simulink model "modello_completo_simulink2017b"  (R2017b)
settings: Solver=VariableStepAuto  StartTime=0.0  StopTime=10  RelTol=1e-3
undefined symbols (not defined in the file): a1, a2, AHRS_bias, AHRS_sample_time, AHRS_var, alpha1, alpha2, c, current, D, dead_zone_limit, DVL_sample_t, DVL_var1, DVL_var2, DVL_var3, gps_sample_t, IMU_sample_time, initial, M, M_inv, n_max, omega, ps_sample_t, ps_sample_t2, ps_var, ps_var2, pylonCenter, pylonRadius, rho, s_data, TAM
libraries: simulink x3
(part 2 of 2)

== system modello_completo_simulink2017b/Vehicle Model/Thrusters/T/Thruster 4 ==
  note: n is the rotational speed of the thruster
      | V is the speed component of the water along the thruster axis
      |
      | n is saturated according to data
      | a dead zone is considered according to data
      | the thruster is characterised by 1st order dynamics (tau = 0.2s)
  n [rad/s] : Inport
  V [m/s] : Inport  Port=2
  Dead Zone : DeadZone  LowerValue=-dead_zone_limit  UpperValue=dead_zone_limit  SaturateOnIntegerOverflow=on
  MATLAB Function : MATLAB Function  TreatAsAtomicUnit=on
  Saturation : Saturate  UpperLimit=n_max  LowerLimit=-n_max
  Transfer Fcn : TransferFcn  Denominator=[0.2 1]
  T i : Outport
  wires:
  V [m/s]/1 -> MATLAB Function/2(V)
  Saturation/1 -> MATLAB Function/1(n)
  Transfer Fcn/1 -> Saturation/1
  Dead Zone/1 -> Transfer Fcn/1
  n [rad/s]/1 -> Dead Zone/1
  MATLAB Function/1(T) -> T i/1

== system modello_completo_simulink2017b/Vehicle Model/Thrusters/T/Thruster 5 ==
  note: n is the rotational speed of the thruster
      | V is the speed component of the water along the thruster axis
      |
      | n is saturated according to data
      | a dead zone is considered according to data
      | the thruster is characterised by 1st order dynamics (tau = 0.2s)
  n [rad/s] : Inport
  V [m/s] : Inport  Port=2
  Dead Zone : DeadZone  LowerValue=-dead_zone_limit  UpperValue=dead_zone_limit  SaturateOnIntegerOverflow=on
  MATLAB Function : MATLAB Function  TreatAsAtomicUnit=on
  Saturation : Saturate  UpperLimit=n_max  LowerLimit=-n_max
  Transfer Fcn : TransferFcn  Denominator=[0.2 1]
  T i : Outport
  wires:
  V [m/s]/1 -> MATLAB Function/2(V)
  Saturation/1 -> MATLAB Function/1(n)
  Transfer Fcn/1 -> Saturation/1
  Dead Zone/1 -> Transfer Fcn/1
  n [rad/s]/1 -> Dead Zone/1
  MATLAB Function/1(T) -> T i/1

== system modello_completo_simulink2017b/Vehicle Model/Thrusters/T/Thruster 6 ==
  note: n is the rotational speed of the thruster
      | V is the speed component of the water along the thruster axis
      |
      | n is saturated according to data
      | a dead zone is considered according to data
      | the thruster is characterised by 1st order dynamics (tau = 0.2s)
  n [rad/s] : Inport
  V [m/s] : Inport  Port=2
  Dead Zone : DeadZone  LowerValue=-dead_zone_limit  UpperValue=dead_zone_limit  SaturateOnIntegerOverflow=on
  MATLAB Function : MATLAB Function  TreatAsAtomicUnit=on
  Saturation : Saturate  UpperLimit=n_max  LowerLimit=-n_max
  Transfer Fcn : TransferFcn  Denominator=[0.2 1]
  T i : Outport
  wires:
  V [m/s]/1 -> MATLAB Function/2(V)
  Saturation/1 -> MATLAB Function/1(n)
  Transfer Fcn/1 -> Saturation/1
  Dead Zone/1 -> Transfer Fcn/1
  n [rad/s]/1 -> Dead Zone/1
  MATLAB Function/1(T) -> T i/1

== system modello_completo_simulink2017b/Vehicle Model/Thrusters/T/Thruster 7 ==
  note: n is the rotational speed of the thruster
      | V is the speed component of the water along the thruster axis
      |
      | n is saturated according to data
      | a dead zone is considered according to data
      | the thruster is characterised by 1st order dynamics (tau = 0.2s)
  n [rad/s] : Inport
  V [m/s] : Inport  Port=2
  Dead Zone : DeadZone  LowerValue=-dead_zone_limit  UpperValue=dead_zone_limit  SaturateOnIntegerOverflow=on
  MATLAB Function : MATLAB Function  TreatAsAtomicUnit=on
  Saturation : Saturate  UpperLimit=n_max  LowerLimit=-n_max
  Transfer Fcn : TransferFcn  Denominator=[0.2 1]
  T i : Outport
  wires:
  V [m/s]/1 -> MATLAB Function/2(V)
  Saturation/1 -> MATLAB Function/1(n)
  Transfer Fcn/1 -> Saturation/1
  Dead Zone/1 -> Transfer Fcn/1
  n [rad/s]/1 -> Dead Zone/1
  MATLAB Function/1(T) -> T i/1

== matlab function modello_completo_simulink2017b/Vehicle Model/Model Vehicle/D ==
  data: ni_r input; F_d output; rho input
function F_d = D_forces(ni_r, rho)
    ni_lin = ni_r(1:3);
    ni_ang = ni_r(4:6);
    a = 0.35;
    b = a;
    c = 0.19;
    A_ab = pi*a*b;      % moto lin lungo z; rotatorio intorno a x e y
    A_bc = pi*b*c;      % moto lin lungo x; rotatorio intorno a z
    A_ac = pi*a*c;      % moto lin lungo y
%     C_d  =  0.0489;
%     D_coeff = -1/2*rho*C_d*diag([A_bc, A_ac, A_ab, A_bc, A_ac, A_ab]);
%     F_d = D_coeff*(abs(ni_r).*ni_r);
    visc = 0.001;       % Pa*s (per una temperatura di 20° e rho = 1030)
    vmax = 0.3;
    Di = 0.7;
    Re = Di/(visc/rho)*vmax; % Re = 2*1e5
    Cd = 0.49;
    rm_z = 4*c/(3*pi);
    rm_xy = 4*a/(3*pi);
    D_lin = -1/2*rho*Cd*diag([A_bc, A_ac, A_ab])*(abs(ni_lin).*ni_lin);
    D_ang = -1/2*rho*Cd*diag([rm_xy^3*A_ab, rm_xy^3*A_ab, rm_z^3*A_bc])*(abs(ni_ang).*ni_ang);
    F_d = [D_lin; D_ang];
end

== matlab function modello_completo_simulink2017b/Vehicle Model/Model Vehicle/C ==
  data: ni_r input; F_c output; M input
function F_c = C(ni_r, M)
    ni = ni_r;
    M11 = M(1:3,1:3);
    M22 = M(4:6,4:6);
    ni1 = ni(1:3);
    ni2 = ni(4:6);
    C11 = zeros(3,3);
    s1 = M11*ni1;
    C12 = - [0 -s1(3) s1(2); s1(3) 0 -s1(1); -s1(2) s1(1) 0];
    C21 = C12;
    s2 = M22*ni2;
    C22 = - [0 -s2(3) s2(2); s2(3) 0 -s2(1); -s2(2) s2(1) 0];
    F_c = [C11 C12; C21 C22]*ni_r;
end

== matlab function modello_completo_simulink2017b/Vehicle Model/Model Vehicle/grav ==
  data: rho input; eta input; F_g output
function F_g = grav(rho, eta)
    eta2 = eta(4:6);
    g = 9.81;   
    a = 0.35;
    b = a;
    c = 0.19;
    massa = 100;
    if eta(3) >= c
       V = 4/3*pi*a*b*c;
    else
       V = 4/3*pi*a*b*c - (pi*a*b/(3*c^2))*((eta(3)-c)^2)*(3*c - abs(eta(3) - c)); 
    end
    W = massa*g;
    B = rho*V*g;
    J = Jac(eta2);
    J1 = J(1:3,1:3);
    J2 = J(4:6,4:6);
    f_g = inv(J1)*[0; 0; W];
    f_b = inv(J1)*[0; 0; -B];
    r_g = [0; 0; 0];
    r_b = [0; 0; -c/2];
    %TODO: inserire un contributo nullo di forza quando siamo a galla (?)
%     if eta(3) < 0
%        F_g = [0; 0; 0; 0; 0; 0];
%     else
    F_g = -[f_g + f_b; cross(r_g,f_g) + cross(r_b,f_b)];
%     end
end

== matlab function modello_completo_simulink2017b/Vehicle Model/Model Vehicle/Kinematic/Jac ==
  data: eta input; J output
function J = Jac(eta)
    eta2 = eta(4:6);
    phi = eta2(1);
    theta = eta2(2);
    psi = eta2(3);
    Rx = [1 0 0; 0 cos(phi) sin(phi); 0 -sin(phi) cos(phi)];
    Ry = [cos(theta) 0 -sin(theta); 0 1 0; sin(theta) 0 cos(theta)];
    Rz = [cos(psi) sin(psi) 0; -sin(psi) cos(psi) 0; 0 0 1];
    J1 = Rz'*Ry'*Rx';
    J2 = [1 sin(phi)*tan(theta) cos(phi)*tan(theta); ...
        0 cos(phi) -sin(phi); ...
        0 sin(phi)/cos(theta) cos(phi)/cos(theta)];
    J = blkdiag(J1, J2);
end

== matlab function modello_completo_simulink2017b/Vehicle Model/Thrusters/T/Thruster 1/MATLAB Function ==
  data: n input; T output; V input; D parameter; omega parameter; a1 parameter; a2 parameter; alpha1 parameter; alpha2 parameter
function T = thrusterModel(n, V, D, omega, a1, a2, alpha1, alpha2)

Va = (1-omega) * V;     % Advancement velocity at the propeller
J0 = Va/(n*D);          % Advancement Coefficient

if J0 > -alpha1/alpha2  % Out of linearity domain (right side)
    T = 0;              % A null generated thrust is assumed
    
elseif J0 < 0           % Out of linearity domain (left side)
    T = a1*abs(n)*n;    % Bollard thrust is assumed

else                    % Within the linearity domain
    T = a1*abs(n)*n - a2*abs(n)*V;
end

== matlab function modello_completo_simulink2017b/Vehicle Model/Thrusters/T/Thruster 2/MATLAB Function ==
  data: n input; T output; V input; D parameter; omega parameter; a1 parameter; a2 parameter; alpha1 parameter; alpha2 parameter
function T = thrusterModel(n, V, D, omega, a1, a2, alpha1, alpha2)

Va = (1-omega) * V;     % Advancement velocity at the propeller
J0 = Va/(n*D);          % Advancement Coefficient

if J0 > -alpha1/alpha2  % Out of linearity domain (right side)
    T = 0;              % A null generated thrust is assumed
    
elseif J0 < 0           % Out of linearity domain (left side)
    T = a1*abs(n)*n;    % Bollard thrust is assumed

else                    % Within the linearity domain
    T = a1*abs(n)*n - a2*abs(n)*V;
end

== matlab function modello_completo_simulink2017b/Vehicle Model/Thrusters/T/Thruster 3/MATLAB Function ==
  data: n input; T output; V input; D parameter; omega parameter; a1 parameter; a2 parameter; alpha1 parameter; alpha2 parameter
function T = thrusterModel(n, V, D, omega, a1, a2, alpha1, alpha2)

Va = (1-omega) * V;     % Advancement velocity at the propeller
J0 = Va/(n*D);          % Advancement Coefficient

if J0 > -alpha1/alpha2  % Out of linearity domain (right side)
    T = 0;              % A null generated thrust is assumed
    
elseif J0 < 0           % Out of linearity domain (left side)
    T = a1*abs(n)*n;    % Bollard thrust is assumed

else                    % Within the linearity domain
    T = a1*abs(n)*n - a2*abs(n)*V;
end

== matlab function modello_completo_simulink2017b/Vehicle Model/Thrusters/T/Thruster 4/MATLAB Function ==
  data: n input; T output; V input; D parameter; omega parameter; a1 parameter; a2 parameter; alpha1 parameter; alpha2 parameter
function T = thrusterModel(n, V, D, omega, a1, a2, alpha1, alpha2)

Va = (1-omega) * V;     % Advancement velocity at the propeller
J0 = Va/(n*D);          % Advancement Coefficient

if J0 > -alpha1/alpha2  % Out of linearity domain (right side)
    T = 0;              % A null generated thrust is assumed
    
elseif J0 < 0           % Out of linearity domain (left side)
    T = a1*abs(n)*n;    % Bollard thrust is assumed

else                    % Within the linearity domain
    T = a1*abs(n)*n - a2*abs(n)*V;
end

== matlab function modello_completo_simulink2017b/Vehicle Model/Thrusters/T/Thruster 5/MATLAB Function ==
  data: n input; T output; V input; D parameter; omega parameter; a1 parameter; a2 parameter; alpha1 parameter; alpha2 parameter
function T = thrusterModel(n, V, D, omega, a1, a2, alpha1, alpha2)

Va = (1-omega) * V;     % Advancement velocity at the propeller
J0 = Va/(n*D);          % Advancement Coefficient

if J0 > -alpha1/alpha2  % Out of linearity domain (right side)
    T = 0;              % A null generated thrust is assumed
    
elseif J0 < 0           % Out of linearity domain (left side)
    T = a1*abs(n)*n;    % Bollard thrust is assumed

else                    % Within the linearity domain
    T = a1*abs(n)*n - a2*abs(n)*V;
end

== matlab function modello_completo_simulink2017b/Vehicle Model/Thrusters/T/Thruster 6/MATLAB Function ==
  data: n input; T output; V input; D parameter; omega parameter; a1 parameter; a2 parameter; alpha1 parameter; alpha2 parameter
function T = thrusterModel(n, V, D, omega, a1, a2, alpha1, alpha2)

Va = (1-omega) * V;     % Advancement velocity at the propeller
J0 = Va/(n*D);          % Advancement Coefficient

if J0 > -alpha1/alpha2  % Out of linearity domain (right side)
    T = 0;              % A null generated thrust is assumed
    
elseif J0 < 0           % Out of linearity domain (left side)
    T = a1*abs(n)*n;    % Bollard thrust is assumed

else                    % Within the linearity domain
    T = a1*abs(n)*n - a2*abs(n)*V;
end

== matlab function modello_completo_simulink2017b/Vehicle Model/Thrusters/T/Thruster 7/MATLAB Function ==
  data: n input; T output; V input; D parameter; omega parameter; a1 parameter; a2 parameter; alpha1 parameter; alpha2 parameter
function T = thrusterModel(n, V, D, omega, a1, a2, alpha1, alpha2)

Va = (1-omega) * V;     % Advancement velocity at the propeller
J0 = Va/(n*D);          % Advancement Coefficient

if J0 > -alpha1/alpha2  % Out of linearity domain (right side)
    T = 0;              % A null generated thrust is assumed
    
elseif J0 < 0           % Out of linearity domain (left side)
    T = a1*abs(n)*n;    % Bollard thrust is assumed

else                    % Within the linearity domain
    T = a1*abs(n)*n - a2*abs(n)*V;
end

== matlab function modello_completo_simulink2017b/Vehicle Model/Model Vehicle/MATLAB Function ==
  data: coord_pylon input; eta input; eta_ecef output
function eta_ecef = nedToEcef(coord_pylon, eta)

    coder.extrinsic('wgs84Ellipsoid');

    coder.extrinsic('ned2geodetic');
    
    eta_pos = eta(1:6);
    wgs84 = wgs84Ellipsoid('meter'); %TODO verificare che esprima le coordinate nello stesso modo dell'ECEF dato in missionB.m
    [eta_pos(1), eta_pos(2)] = ned2geodetic(eta(1), eta(2), eta(3), coord_pylon(1), coord_pylon(2), coord_pylon(3), wgs84,'degrees');
    
    eta_pos(3) = eta(3);
    eta_pos(4:6) = eta_pos(4:6);
    
    eta_ecef = eta_pos;
    
end

== matlab function modello_completo_simulink2017b/Vehicle Model/MATLAB Function ==
  data: eta input; ni_c output; current input
function ni_c = current_ned2body(eta, current)
    eta2 = eta(4:6)*pi/180;     % eta2 espresso in radianti
    ni_c = Jac(eta2)'*current;
end

== matlab function modello_completo_simulink2017b/Vehicle Model/Thrusters/T/MATLAB Function ==
  data: ni input; v_th output
function v_th = thrusters(ni)
p1 = [-0.35 -0.25 0]';
p2 = [-0.35 0.25 0]';
p3 = [-0.25 -0.35 0]';
p4 = [0.25 0.35 0]';
p5 = [-0.25 -0.25 -0.19]';
p6 = [-0.25 0.25 -0.19]';
p7 = [0.25 0 -0.19]';

t1 = [1 0 0]';
t2 = t1;
t3 = [0 1 0]';
t4 = -t3;
t5 = [0 0 1]';
t6 = t5;
t7 = t5;

v_lin = ni(1:3);
v_ang = ni(4:6);

vp1 = v_lin + cross(v_ang, p1);
vp2 = v_lin + cross(v_ang, p2);
vp3 = v_lin + cross(v_ang, p3);
vp4 = v_lin + cross(v_ang, p4);
vp5 = v_lin + cross(v_ang, p5);
vp6 = v_lin + cross(v_ang, p6);
vp7 = v_lin + cross(v_ang, p7);

v1 = vp1'*t1;
v2 = vp2'*t2;
v3 = vp3'*t3;
v4 = vp4'*t4;
v5 = vp5'*t5;
v6 = vp6'*t6;
v7 = vp7'*t7;

v_th = [ v1 v2 v3 v4 v5 v6 v7]';
end

== matlab function modello_completo_simulink2017b/Vehicle Model/Thrusters/saturation_tau ==
  data: tau input; tau_sat output; eta input
function tau_sat = sat_tau(tau, eta)
    tau_sat = [0;0;0;0;0;0];
    tau_sat = tau;

    if eta(3) < 0.1 %semiasse c
        tau_sat(3) = 0;
    end
    
end

== matlab function modello_completo_simulink2017b/Navigation/Geodetic to NED/MATLAB Function2 ==
  data: GPS_geodetic input; GPS_flag input; GPS_NED output; depth input; pylonCenter parameter
function GPS_NED = Geo2NED(GPS_geodetic, GPS_flag, depth, pylonCenter)

if GPS_flag == 0
    GPS_NED = [0;0;0];
    return
end

%% variabili

phi = GPS_geodetic(1);
lambda = GPS_geodetic(2);
h = -depth;

phi_pyl = pylonCenter(1) * pi/180;    % GPS_geodetic_origin 
lambda_pyl = pylonCenter(2) * pi/180;

% r_e = 6378137;
% epsilon = 0.08181919;
% N = r_e / (sqrt(1 - epsilon^2 * (sin(phi))^2));
% N_pyl = r_e / (sqrt(1 - epsilon^2 * (sin(phi_pyl))^2));
% 
% eta_ECEF_origin = zeros(3,1);
% eta_ECEF_origin = [(N_pyl + h) * cos(phi_pyl) * cos(lambda_pyl);
%                    (N_pyl + h) * cos(phi_pyl) * sin(lambda_pyl);
%                    (N_pyl*(1-epsilon^2) + h) * sin(phi_pyl)];
% 
% %% da geodetic a ECEF
% eta_ECEF_P = zeros(3,1);
% eta_ECEF_P = [(N + h) * cos(phi) * cos(lambda);
%               (N + h) * cos(phi) * sin(lambda);
%               (N*(1-epsilon^2) + h) * sin(phi)];
% 
% %% da ECEF a NED
% 
% R_ECEF_NED = [-sin(phi_pyl)*cos(lambda_pyl),    -sin(phi_pyl)*sin(lambda_pyl),  cos(phi_pyl);   % matrice "C" 3x3
%               -sin(lambda_pyl),                 cos(lambda_pyl),                0;
%               -cos(phi_pyl)*cos(lambda_pyl),    -cos(phi_pyl)*sin(lambda_pyl),  -sin(phi_pyl)];
% 
% R_ECEF_NED_2 = R_ECEF_NED(1:2,:);   % matrice "C" 2x3
% eta_NED_GPS = zeros(2,1);
% eta_ECEF = (eta_ECEF_P - eta_ECEF_origin);
% 
% eta_NED_GPS = R_ECEF_NED_2 * eta_ECEF;   % solo gli elementi x,y di eta
coder.extrinsic('wgs84Ellipsoid');

coder.extrinsic('geodetic2ned');
    
[x_gps2, y_gps2, z_gps2] = geodetic2ned(phi, lambda, -depth, phi_pyl, lambda_pyl, 0, wgs84Ellipsoid, 'radians');
eta_NED_GPS = [x_gps2; y_gps2];
GPS_NED = zeros(3,1);
GPS_NED(1) = eta_NED_GPS(1);
GPS_NED(2) = eta_NED_GPS(2);
GPS_NED(3) = GPS_flag;
                                                            % uscita in radianti

== matlab function modello_completo_simulink2017b/Navigation/MATLAB Function ==
  data: flag_depth input; flag_AHRS input; error_flag output; flag_DVL input; flag_sonar input
function error_flag = fcn(flag_depth, flag_AHRS, flag_DVL, flag_sonar)
flag_ahrs = flag_AHRS(1) & flag_AHRS(2) & flag_AHRS(3);
error_flag = flag_depth & flag_ahrs & flag_DVL & flag_sonar;
%se vi è un errore vale 0

== matlab function modello_completo_simulink2017b/Navigation/MATLAB Function7 ==
  data: eta2 output; lin_acc input; nu2 output; ang_vel input; orientation input
function [eta2, nu2]= AHRS_signals(lin_acc, ang_vel, orientation)
acc = lin_acc(1:3);
nu2 = ang_vel(1:3);
eta2 = orientation(1:3);

== matlab function modello_completo_simulink2017b/Navigation/MATLAB Function8 ==
  data: dvl input; velocity_est output; flag_DVL output
function [velocity_est, flag_DVL] = DVL_signals(dvl)
% y = lowpass(u, 0.01);
flag_DVL = dvl(4);
velocity_est = dvl(1:3);

== matlab function modello_completo_simulink2017b/Navigation/NED to Geodetic/MATLAB Function1 ==
  data: eta_NED input; eta_geodetic output; depth input; pylonCenter parameter
function eta_geodetic = NED2Geo(eta_NED, depth, pylonCenter)
coder.extrinsic('fcn_NED2GeoN');
eta_geodetic = [0; 0];
eta_geodetic = fcn_NED2GeoN(eta_NED, depth, pylonCenter);
end

== matlab function modello_completo_simulink2017b/Navigation/Relative estiamtion/Sonar trigger/MATLAB Function ==
  data: sonar input; sum input; pulse output; prev output
function [pulse, prev] = fcn(sonar, sum)


if all(sum) == 0
    pulse = 0;
else
    pulse = 1;
end

prev = sonar;

== matlab function modello_completo_simulink2017b/Navigation/Relative estiamtion/Subsystem/MATLAB Function9 ==
  data: sonar input; orientation input; distance output; alpha output; flag_sonar output; pylonRadius parameter
function [distance, alpha, flag_sonar] = relative_values(sonar, orientation, pylonRadius)
coder.extrinsic('fcn_sonar');
distance = 0;
alpha = 0;
flag_sonar = 0;
[distance, alpha, flag_sonar] = fcn_sonar(sonar, orientation, pylonRadius);
end

== matlab function modello_completo_simulink2017b/Navigation/Subsystem/EKF/EKF_depth/Correzione ==
  data: P_depth output; P_depth input; hat_depth input; depth_meas input; hat_depth output; flag_depth output; R parameter
function [P_depth, hat_depth, flag_depth]  = EKF_depth(P_depth, hat_depth, depth_meas, R)

%% Inizializzazione

DT = 1/50;                           % frequenza profondimetro = 50 Hz

%% EKF



% Correzione
z_tilde = depth_meas(1) - hat_depth;
H = 1;
S = H * P_depth * H' + R(3,3);

K = P_depth * H' * S^(-1);

hat_depth = hat_depth + K * z_tilde;   
P_depth   = (1 - K * H) * P_depth;  

    
flag_depth = depth_meas(2);

== matlab function modello_completo_simulink2017b/Navigation/Subsystem/EKF/EKF_depth/Predizione ==
  data: P_depth output; P_depth input; hat_depth input; dT input; hat_depth output; orientation input; dvl input; init_depth input; P0_depth input; ahrs_flag input; Q parameter
function [P_depth, hat_depth]  = EKF_depth(P_depth, hat_depth, dT, orientation, dvl, init_depth, P0_depth, ahrs_flag, Q)

%% Inizializzazione
                     % [s]  depth period
dvl_flag = dvl(4);

%coder.extrinsic('Lk_func');

if hat_depth == 0
    hat_depth = init_depth;
    P_depth = P0_depth;
end

if (ahrs_flag && dvl_flag) == 1

    phi    =  orientation(1);  % roll
    theta  =  orientation(2);  % pitch
    psi_    =  orientation(3);  % yaw
    vel    = [dvl(1); dvl(2); dvl(3)];
    J=zeros(3,3);
    Lk=zeros(3,6);
    
%    [J, Lk] = Lk_func(dT, psi, theta, psi, vel);

J = [ cos(psi_)*cos(theta), cos(psi_)*sin(phi)*sin(theta) - cos(phi)*sin(psi_), sin(phi)*sin(psi_) + cos(phi)*cos(psi_)*sin(theta);
       cos(theta)*sin(psi_), cos(phi)*cos(psi_) + sin(phi)*sin(psi_)*sin(theta), cos(phi)*sin(psi_)*sin(theta) - cos(psi_)*sin(phi);
         -sin(theta),                                cos(theta)*sin(phi),                                cos(phi)*cos(theta)];
     
%J = eval(subs(J1, {phi, theta, psi_}, {phi, theta, psi_}));

x = dvl(1);
y = dvl(2);
z = dvl(3);
n_ahrs1 = 0;
n_ahrs2 = 0;
n_ahrs3 = 0;

Lk = [  dT*(y*(sin(n_ahrs1 + phi)*sin(n_ahrs3 + psi_) + cos(n_ahrs1 + phi)*cos(n_ahrs3 + psi_)*sin(n_ahrs2 + theta)) + z*(cos(n_ahrs1 + phi)*sin(n_ahrs3 + psi_) - cos(n_ahrs3 + psi_)*sin(n_ahrs1 + phi)*sin(n_ahrs2 + theta))), dT*(z*cos(n_ahrs1 + phi)*cos(n_ahrs3 + psi_)*cos(n_ahrs2 + theta) - x*cos(n_ahrs3 + psi_)*sin(n_ahrs2 + theta) + y*cos(n_ahrs3 + psi_)*cos(n_ahrs2 + theta)*sin(n_ahrs1 + phi)), -dT*(y*(cos(n_ahrs1 + phi)*cos(n_ahrs3 + psi_) + sin(n_ahrs1 + phi)*sin(n_ahrs3 + psi_)*sin(n_ahrs2 + theta)) - z*(cos(n_ahrs3 + psi_)*sin(n_ahrs1 + phi) - cos(n_ahrs1 + phi)*sin(n_ahrs3 + psi_)*sin(n_ahrs2 + theta)) + x*cos(n_ahrs2 + theta)*sin(n_ahrs3 + psi_)), dT*cos(n_ahrs3 + psi_)*cos(n_ahrs2 + theta), -dT*(cos(n_ahrs1 + phi)*sin(n_ahrs3 + psi_) - cos(n_ahrs3 + psi_)*sin(n_ahrs1 + phi)*sin(n_ahrs2 + theta)),  dT*(sin(n_ahrs1 + phi)*sin(n_ahrs3 + psi_) + cos(n_ahrs1 + phi)*cos(n_ahrs3 + psi_)*sin(n_ahrs2 + theta));
 -dT*(y*(cos(n_ahrs3 + psi_)*sin(n_ahrs1 + phi) - cos(n_ahrs1 + phi)*sin(n_ahrs3 + psi_)*sin(n_ahrs2 + theta)) + z*(cos(n_ahrs1 + phi)*cos(n_ahrs3 + psi_) + sin(n_ahrs1 + phi)*sin(n_ahrs3 + psi_)*sin(n_ahrs2 + theta))), dT*(z*cos(n_ahrs1 + phi)*cos(n_ahrs2 + theta)*sin(n_ahrs3 + psi_) - x*sin(n_ahrs3 + psi_)*sin(n_ahrs2 + theta) + y*cos(n_ahrs2 + theta)*sin(n_ahrs1 + phi)*sin(n_ahrs3 + psi_)),  dT*(z*(sin(n_ahrs1 + phi)*sin(n_ahrs3 + psi_) + cos(n_ahrs1 + phi)*cos(n_ahrs3 + psi_)*sin(n_ahrs2 + theta)) - y*(cos(n_ahrs1 + phi)*sin(n_ahrs3 + psi_) - cos(n_ahrs3 + psi_)*sin(n_ahrs1 + phi)*sin(n_ahrs2 + theta)) + x*cos(n_ahrs3 + psi_)*cos(n_ahrs2 + theta)), dT*cos(n_ahrs2 + theta)*sin(n_ahrs3 + psi_),  dT*(cos(n_ahrs1 + phi)*cos(n_ahrs3 + psi_) + sin(n_ahrs1 + phi)*sin(n_ahrs3 + psi_)*sin(n_ahrs2 + theta)), -dT*(cos(n_ahrs3 + psi_)*sin(n_ahrs1 + phi) - cos(n_ahrs1 + phi)*sin(n_ahrs3 + psi_)*sin(n_ahrs2 + theta));
                                                                                                                                dT*(y*cos(n_ahrs1 + phi)*cos(n_ahrs2 + theta) - z*cos(n_ahrs2 + theta)*sin(n_ahrs1 + phi)),                                                            -dT*(x*cos(n_ahrs2 + theta) + z*cos(n_ahrs1 + phi)*sin(n_ahrs2 + theta) + y*sin(n_ahrs1 + phi)*sin(n_ahrs2 + theta)),                                                                                                                                                                                                                                                                      0,                    -dT*sin(n_ahrs2 + theta),                                                                 dT*cos(n_ahrs2 + theta)*sin(n_ahrs1 + phi),                                                                 dT*cos(n_ahrs1 + phi)*cos(n_ahrs2 + theta)];
                                                                                                                            
%Lk = eval(subs(L, {dT, phi, theta, psi_, n_ahrs1, n_ahrs2, n_ahrs3, x, y, z}, {DT, phi, theta, psi, 0, 0, 0, dvl(1), dvl(2), dvl(3)}));


    %% EKF
    % Predizione
    hat_depth = hat_depth + dT * J(3,[1,2,3]) *vel;        
    P_depth   = P_depth   + Lk(3, [3,6]) * Q([3,6], [3,6]) * Lk(3, [3,6])';      %colonne 3 e 6

end

== matlab function modello_completo_simulink2017b/Navigation/Subsystem/EKF/EKF_position/Correzione  ==
  data: prev_pos output; prev_pos input; P_pos input; hat_pos input; P_pos output; meas_pos input; hat_pos output; GPS_flag input; R parameter
function [prev_pos, P_pos, hat_pos] = EKF_pos(prev_pos, P_pos, hat_pos,  meas_pos, GPS_flag, R)

% Prendiamo in ingresso la posizione stimata al passo precedente e la predizione P,
% la posizione stimata dal GPS, tutti i valori dell'AHRS ed il DVL.


%%Inizializzazione      
H    =  eye(2);


%% EKF: Correzione

if all(meas_pos - prev_pos) ~= 0 && GPS_flag == 1               %se il flag=1 il GPS sta funzionando

    z_tilde = meas_pos - hat_pos;

    S = H * P_pos * H' + R([1,2],[1,2]);

    K = P_pos * H' * S^(-1);

    hat_pos = hat_pos + K * z_tilde;   
    P_pos = (eye(2) - K * H) * P_pos;  
    
    prev_pos = meas_pos;
    
else
    
    %P_pos   = P_pos;
    %hat_pos = hat_pos;
    %prev_pos = prev_pos;
    
end

== matlab function modello_completo_simulink2017b/Navigation/Subsystem/EKF/EKF_position/Predizione ==
  data: P_pos input; hat_pos input; dT input; P_pos output; hat_pos output; orientation input; dvl input; ahrs_flag input; init_pos input; P0_pos input; Q parameter
function [P_pos, hat_pos]  = EKF_pos(P_pos, hat_pos, dT, orientation, dvl, ahrs_flag, init_pos, P0_pos, Q)

dvl_flag = dvl(4);

%coder.extrinsic('Lk_func');

if all(hat_pos) == 0
    hat_pos = init_pos;
    P_pos = P0_pos;
end

if (ahrs_flag && dvl_flag) == 1

    phi    =  orientation(1);  % roll
    theta  =  orientation(2);  % pitch
    psi_    =  orientation(3);  % yaw
    vel    = [dvl(1); dvl(2); dvl(3)];
    J=zeros(3,3);
    Lk=zeros(3,6);
    
    %[J, Lk] = Lk_func(dT, psi, theta, psi, vel);

    
    J = [ cos(psi_)*cos(theta), cos(psi_)*sin(phi)*sin(theta) - cos(phi)*sin(psi_), sin(phi)*sin(psi_) + cos(phi)*cos(psi_)*sin(theta);
       cos(theta)*sin(psi_), cos(phi)*cos(psi_) + sin(phi)*sin(psi_)*sin(theta), cos(phi)*sin(psi_)*sin(theta) - cos(psi_)*sin(phi);
         -sin(theta),                                cos(theta)*sin(phi),                                cos(phi)*cos(theta)];
     
%J = eval(subs(J1, {phi, theta, psi_}, {phi, theta, psi_}));

x = dvl(1);
y = dvl(2);
z = dvl(3);
n_ahrs1 = 0;
n_ahrs2 = 0;
n_ahrs3 = 0;


Lk = [  dT*(y*(sin(n_ahrs1 + phi)*sin(n_ahrs3 + psi_) + cos(n_ahrs1 + phi)*cos(n_ahrs3 + psi_)*sin(n_ahrs2 + theta)) + z*(cos(n_ahrs1 + phi)*sin(n_ahrs3 + psi_) - cos(n_ahrs3 + psi_)*sin(n_ahrs1 + phi)*sin(n_ahrs2 + theta))), dT*(z*cos(n_ahrs1 + phi)*cos(n_ahrs3 + psi_)*cos(n_ahrs2 + theta) - x*cos(n_ahrs3 + psi_)*sin(n_ahrs2 + theta) + y*cos(n_ahrs3 + psi_)*cos(n_ahrs2 + theta)*sin(n_ahrs1 + phi)), -dT*(y*(cos(n_ahrs1 + phi)*cos(n_ahrs3 + psi_) + sin(n_ahrs1 + phi)*sin(n_ahrs3 + psi_)*sin(n_ahrs2 + theta)) - z*(cos(n_ahrs3 + psi_)*sin(n_ahrs1 + phi) - cos(n_ahrs1 + phi)*sin(n_ahrs3 + psi_)*sin(n_ahrs2 + theta)) + x*cos(n_ahrs2 + theta)*sin(n_ahrs3 + psi_)), dT*cos(n_ahrs3 + psi_)*cos(n_ahrs2 + theta), -dT*(cos(n_ahrs1 + phi)*sin(n_ahrs3 + psi_) - cos(n_ahrs3 + psi_)*sin(n_ahrs1 + phi)*sin(n_ahrs2 + theta)),  dT*(sin(n_ahrs1 + phi)*sin(n_ahrs3 + psi_) + cos(n_ahrs1 + phi)*cos(n_ahrs3 + psi_)*sin(n_ahrs2 + theta));
 -dT*(y*(cos(n_ahrs3 + psi_)*sin(n_ahrs1 + phi) - cos(n_ahrs1 + phi)*sin(n_ahrs3 + psi_)*sin(n_ahrs2 + theta)) + z*(cos(n_ahrs1 + phi)*cos(n_ahrs3 + psi_) + sin(n_ahrs1 + phi)*sin(n_ahrs3 + psi_)*sin(n_ahrs2 + theta))), dT*(z*cos(n_ahrs1 + phi)*cos(n_ahrs2 + theta)*sin(n_ahrs3 + psi_) - x*sin(n_ahrs3 + psi_)*sin(n_ahrs2 + theta) + y*cos(n_ahrs2 + theta)*sin(n_ahrs1 + phi)*sin(n_ahrs3 + psi_)),  dT*(z*(sin(n_ahrs1 + phi)*sin(n_ahrs3 + psi_) + cos(n_ahrs1 + phi)*cos(n_ahrs3 + psi_)*sin(n_ahrs2 + theta)) - y*(cos(n_ahrs1 + phi)*sin(n_ahrs3 + psi_) - cos(n_ahrs3 + psi_)*sin(n_ahrs1 + phi)*sin(n_ahrs2 + theta)) + x*cos(n_ahrs3 + psi_)*cos(n_ahrs2 + theta)), dT*cos(n_ahrs2 + theta)*sin(n_ahrs3 + psi_),  dT*(cos(n_ahrs1 + phi)*cos(n_ahrs3 + psi_) + sin(n_ahrs1 + phi)*sin(n_ahrs3 + psi_)*sin(n_ahrs2 + theta)), -dT*(cos(n_ahrs3 + psi_)*sin(n_ahrs1 + phi) - cos(n_ahrs1 + phi)*sin(n_ahrs3 + psi_)*sin(n_ahrs2 + theta));
                                                                                                                                dT*(y*cos(n_ahrs1 + phi)*cos(n_ahrs2 + theta) - z*cos(n_ahrs2 + theta)*sin(n_ahrs1 + phi)),                                                            -dT*(x*cos(n_ahrs2 + theta) + z*cos(n_ahrs1 + phi)*sin(n_ahrs2 + theta) + y*sin(n_ahrs1 + phi)*sin(n_ahrs2 + theta)),                                                                                                                                                                                                                                                                      0,                    -dT*sin(n_ahrs2 + theta),                                                                 dT*cos(n_ahrs2 + theta)*sin(n_ahrs1 + phi),                                                                 dT*cos(n_ahrs1 + phi)*cos(n_ahrs2 + theta)];
                                                                                                                            
%Lk = eval(subs(L, {dT, phi, theta, psi_, n_ahrs1, n_ahrs2, n_ahrs3, x, y, z}, {DT, phi, theta, psi, 0, 0, 0, dvl(1), dvl(2), dvl(3)}));


      %% EKF: Predizione

    hat_pos  =  hat_pos + dT * J([1,2],[1,2,3]) * vel;        
    P_pos    =  P_pos + Lk([1,2], [1,2,4,5]) * Q([1,2,4,5],[1,2,4,5]) * Lk([1,2], [1,2,4,5])';       %Lk           

    
end

== matlab function modello_completo_simulink2017b/Navigation/Subsystem/Trigger & Init/Depth trigger/MATLAB Function ==
  data: count input; count output; dT output; depth input; sum input; pulse output; prev output
function [count, dT, pulse, prev] = fcn(count, depth, sum)

dT = 0;
    

if sum == 0
    pulse = 0;
    count = count + 1;
else
    pulse = 1;
    dT = count * (1/200);
    count = 0;
end

prev = depth;

== matlab function modello_completo_simulink2017b/Navigation/Subsystem/Trigger & Init/Initialization/MATLAB Function1 ==
  data: init_counter output; init_counter input; gps input; pulse output; init_pos output; P0_pos output; init_depth output; P0_depth output; prev output; depth input; diff input; store_gps input; gps_store output; store_depth input; depth_store output; maintain_count input; maintain_count output
function [init_counter, pulse, init_pos, P0_pos, init_depth, P0_depth, prev, gps_store, depth_store, maintain_count] = fcn_init(init_counter, gps, depth, diff, store_gps, store_depth, maintain_count)

pulse = 0;
N = 5;
gps_store = store_gps;
depth_store = store_depth;
init_pos = zeros(2,1);
P0_pos = zeros(2);
init_depth = 0;
P0_depth = 0;
coder.extrinsic('init_position');


if all(diff) ~= 0 && init_counter < N
    
    init_counter = init_counter + 1;
    gps_store(1, init_counter) = gps(1);
    gps_store(2, init_counter) = gps(2);
    pulse = 0;
    depth_store(init_counter) = depth;
    
elseif init_counter < N

    init_counter = init_counter;
    pulse = 0;
    
elseif init_counter == N
   
    [init_pos, P0_pos, init_depth, P0_depth] = init_position(store_gps, store_depth, N); 
    pulse = 1;
    init_counter = init_counter + 1;
    
elseif maintain_count < N^2*N^2
    
    [init_pos, P0_pos, init_depth, P0_depth] = init_position(store_gps, store_depth, N); 
    maintain_count = maintain_count + 1;
    pulse = 1;
    
else 
    
    pulse = 1;
   
end


prev = gps;

== matlab function modello_completo_simulink2017b/Env. & Sensor Model/AHRS SENSOR/    ==
  data: ni_1 input; ni_1_dot input; lin_acc output; ang_vel output; m output; ni_2 input; eta_2 input; eta_2_dot input
function [lin_acc, ang_vel, m] = IMU(ni_1, ni_1_dot, ni_2, eta_2, eta_2_dot)

% questa funzione, partendo dalle informazioni cinematiche dell' AUV
% restituisce in output delle misure di accelerazione, velocità angolare
% e campo magnetico locale


% definisco R^T
% R = Rz(psi)*Ry(theta)*Rx(phi);

% yaw = psi; pitch = theta; roll = phi;

phi = eta_2(1);
theta = eta_2(2);
psi = eta_2(3);

R = [cos(psi)*cos(theta) cos(psi)*sin(theta)*sin(phi)-sin(psi)*cos(phi) cos(psi)*sin(theta)*cos(phi)+sin(psi)*sin(phi);
     sin(psi)*cos(theta) sin(psi)*sin(theta)*sin(phi)+cos(psi)*cos(phi) sin(psi)*sin(theta)*cos(phi)-cos(psi)*sin(phi);
    -sin(theta) cos(theta)*sin(phi) cos(theta)*cos(phi)];

% Rx_phi = [1 0 0; 0 cos(phi) sin(phi); 0 -sin(phi) cos(phi)];
% Ry_theta = [cos(theta) 0 -sin(theta); 0 1 0; sin(theta) 0 cos(theta)];
% Rz_psi = [cos(psi) sin(psi) 0; -sin(psi) cos(psi) 0; 0 0 1];

% R = Rz_psi'*Ry_theta'*Rx_phi;

% Definisco la matrice Jacobiana
 
%J_2 = [1 sin(phi)*tan(theta) cos(phi)*tan(theta);
%       0 cos(phi) -sin(phi);
%       0 sin(phi)/cos(theta) cos(phi)/cos(theta)];
  
% accelerometro

g = [0 0 9.82]; % [m/s^2]
 
%lin_acc = J_1' * (eta_1_ddot - g);  
 
% eta_1_ddot = J_1 * ni_1_dot + J_1_dot * ni_1

dphi = eta_2_dot(1);
dtheta = eta_2_dot(2);
dpsi = eta_2_dot(3);


J_1_dot = [-dtheta*(sin(theta)*cos(psi)) - dpsi*(sin(psi)*cos(theta)), ...
           dphi*(sin(psi)*sin(phi) + cos(psi)*sin(theta)*cos(phi)) + dtheta*(cos(psi)*cos(theta)*sin(phi)) - dpsi*(cos(psi)*cos(phi) + sin(psi)*sin(theta)*sin(phi)), ... 
           dphi*(sin(psi)*cos(phi) - cos(psi)*sin(theta)*sin(phi)) + dtheta*(cos(psi)*cos(theta)*cos(phi)) + dpsi*(cos(psi)*sin(phi) - sin(psi)*sin(theta)*cos(phi)); ...
          -dtheta*(sin(theta)*sin(psi)) + dpsi*(cos(psi)*cos(theta)), ...
           dphi*(-cos(psi)*sin(phi) + sin(psi)*sin(theta)*cos(phi)) + dtheta*(sin(psi)*cos(theta)*sin(phi)) + dpsi*(-sin(psi)*cos(phi) + cos(psi)*sin(theta)*sin(phi)), ... 
          -dphi*(cos(psi)*cos(phi) + sin(psi)*sin(theta)*sin(phi)) + dtheta*(sin(psi)*cos(theta)*cos(phi)) + dpsi*(sin(psi)*sin(phi) + cos(psi)*sin(theta)*cos(phi)); ...
          -dtheta*(cos(theta)), ...
           dphi*(cos(theta)*cos(phi)) - dtheta*(sin(theta)*sin(phi)), ...
          -dphi*(cos(theta)*sin(phi)) - dtheta*(sin(theta)*cos(phi))];

% J_1 = R;      

eta_1_ddot = R * ni_1_dot + J_1_dot * ni_1;

lin_acc = R' * (eta_1_ddot - g');
 
 
 %  giroscopio
 
 % se mi fosse stata fornita la eta_2_dot (espressa in terna NED, globale) la
 % misura del giroscopio sarebbe stata:
 
 %ang_vel = inv(J_2) * eta_2_dot;
 
 %avendo a disposizione in ingresso l'accelerazione in terna Body, la
 %misura della velocità angolare sarà:
 
 ang_vel = ni_2;
 
 % magnetometro ( campo magnetico terrestre espresso in terna NED)
 
 
% gaussian =  normrnd([0 0 0], [0.00131, 0.00094, 0.00157]);
% gaussian = incertezza dell'intensità del campo magnetico 
% calcolata su: https://www.ngdc.noaa.gov/geomag/calculators/magcalc.shtml#igrfwmm

 m_e = [0.238836 -0.010851 0.392423]'; % + gaussian';
 
 m = R' * m_e;
 
end

== matlab function modello_completo_simulink2017b/Env. & Sensor Model/DVL SENSOR/MATLAB Function ==
  data: ni input; niDVL output; c parameter
function niDVL = traslation(ni, c)
S = [0,-ni(6),ni(5); 
    ni(6),0,-ni(4); 
    -ni(5),ni(4),0];
p = [0;0;c];
niDVL = ni(1:3,1)+S*p;

== matlab function modello_completo_simulink2017b/Env. & Sensor Model/DVL SENSOR/MATLAB Function2 ==
  data: v input; flag output
%Calcolo modulo della velocità, l'angolo che forma il vettore velocità con
%l'asse z (phi) e l'angolo che la proiezione della velocità sul piano xy
%forma con l'asse x (theta).
function flag  = vel_module(v)
mod = sqrt((v(1))^2+(v(2))^2+(v(3))^2);

%Da datasheet, se la velocità è superiore ai 9 m/s il sensore non funziona bene
if mod > 9
    flag = 0;
else
    flag = 1;
end
end

== matlab function modello_completo_simulink2017b/Env. & Sensor Model/Pressure sensor/MATLAB Function ==
  data: h input; p output
function p = pressure(h)
g = 9.81;   %accelerazione gravitazionale
rho = 1030;
p = rho*g*h;
end

== matlab function modello_completo_simulink2017b/Env. & Sensor Model/Pressure sensor/MATLAB Function1 ==
  data: p input; h output
function h = depth(p)
rho = 1030;
g = 9.81;
h = p/(rho*g);
end

== matlab function modello_completo_simulink2017b/Env. & Sensor Model/Pressure sensor/MATLAB Function2 ==
  data: h input; p output; rho parameter
function p = pressure(h, rho)
g = 9.81;   %accelerazione gravitazionale
p = rho*g*h;
end

== matlab function modello_completo_simulink2017b/Env. & Sensor Model/Pressure sensor/MATLAB Function3 ==
  data: p input; h output; rho parameter; c parameter
function h = depth(p, rho, c)
g = 9.81;
h = p/(rho*g)+c;  %the pressure sensor is installed on the bottom of the AUV, along the z axis
end

== matlab function modello_completo_simulink2017b/Env. & Sensor Model/GPS_SENSOR/NED2Geodetic ==
  data: depth input; u input; data_GDT output; enableGps input; pylonCenter parameter
function data_GDT= fcn(depth, u, enableGps, pylonCenter)

lat_origin = pylonCenter(1);
lon_origin= pylonCenter(2);
h_origin = pylonCenter(3);

xNorth = u(1);
yEast = u(2);

if enableGps==1
    [lat,lon, h] = ned2geodeticS(xNorth, yEast, depth, lat_origin, lon_origin, h_origin);
else
    lat=NaN;
    lon=NaN;
end

data_GDT = [lat, lon];

== matlab function modello_completo_simulink2017b/Env. & Sensor Model/GPS_SENSOR/Threshold ==
  data: depth output; x_out output; x_in input; y_out output; y_in input; h_in input; flag_enable_gps output; gpsThreshold parameter
function [depth, x_out, y_out, flag_enable_gps] = fcn(x_in, y_in, h_in, gpsThreshold)


if (h_in > gpsThreshold) % gps does not work
    flag_enable_gps=0;
    x_in = NaN;
    y_in = NaN;
else % ok gps work 
    flag_enable_gps=1;
end

x_out=x_in;
y_out=y_in;
depth=h_in;

== matlab function modello_completo_simulink2017b/Env. & Sensor Model/Sonar sensor/MATLAB Function ==
  data: xNorth input; s output; yEast input; zDown input; roll input; pitch input; yaw input; pylonRadius parameter; s_data parameter
function s = Sonar_ideal(xNorth,yEast,zDown,roll,pitch,yaw,pylonRadius, s_data)

coder.extrinsic('Sonar_id');

s_data.num = 5;
s = zeros(s_data.num,1);

s = Sonar_id(xNorth,yEast,zDown,roll,pitch,yaw,pylonRadius,s_data);

== matlab function modello_completo_simulink2017b/Env. & Sensor Model/Sonar sensor/MATLAB Function1 ==
  data: s_in input; s_out output; depth input; error input; flag output; s_data parameter
function [s_out,flag] = Sonar_lim(s_in,depth,error,s_data)
%SONAR_lim
%     [s_out,flag] = Sonar_id[s,error]
%
% Returns the sonar output considering the sensors limitations, but not
% taking into account the bias and error.
%
% flag signals that the corresponding sensor output is affected by
% problems:
% flag += 0     ==>     No errors
% flag += 1     ==>     Under minimum detectable range
% flag += 2     ==>     Over maximum detectable range
% flag += 4     ==>     Over maximum depth
% flag += 8     ==>     Other errors
%
% error is a boolean variable which, when true, sets the flag to += 8

s_data.num = 5;

flag = zeros(s_data.num,1);

s_out = s_in;

for i=1:s_data.num
    if s_in(i) < s_data.minrng
        flag(i) = flag(i)+1;
        s_out(i) = s_data.minrng;
    end
    
    if s_in(i) > s_data.maxrng
        flag(i) = flag(i)+2;
        s_out(i) = NaN;
    end
    
    if depth > s_data.maxdpt
        flag(i) = flag(i)+4;
        s_out(i) = NaN;
    end
    
    if error(i) > 0
        flag(i) = flag(i) + error(i);
        s_out(i) = NaN;
    end
end

end

== matlab function modello_completo_simulink2017b/Env. & Sensor Model/draw env/MATLAB Function ==
  data: enable_from_simulink input; u input
function environment(enable_from_simulink, u)

auvCoordinates=[u(1), u(2), u(3)];

coder.extrinsic('draw_movement');

if (enable_from_simulink == 1)
    draw_movement(auvCoordinates)
end

== matlab function modello_completo_simulink2017b/Env. & Sensor Model/geodetic2NED1 ==
  data: x output; u input; y output; z output; pylonCenter parameter
function [x, y, z] = fcn(u, pylonCenter)


lat_origin = pylonCenter(1);
lon_origin= pylonCenter(2);
h_origin = pylonCenter(3);

lat=u(1);
lon=u(2);
h=u(3);


[xNorth, yEast, zDown] = geodetic2nedS(lat, lon, h, lat_origin, lon_origin, h_origin);

x = xNorth;
y = yEast;
z = h;
